simulink model "JIC"  (R2021b)
settings: Solver=ode3  StartTime=0.0  StopTime=10  FixedStep=.002  RelTol=1e-3  EnableMultiTasking=on
libraries: slpidlib x1
settings Model: ExtModeTrigDuration=10000  Creator=smascaro  LastModifiedBy=zorto
settings SolverCC: AlgebraicLoopSolver=TrustRegion  PositivePriorityOrder=on
settings DataIOCC: SaveFormat=Array  SignalLoggingSaveFormat=ModelDataLogs  SaveOutput=off  SaveTime=off  ReturnWorkspaceOutputs=off
settings OptimizationCC: ExpressionDepthLimit=2147483647  InitFltsAndDblsToZero=on  LifeSpan=inf
settings DebuggingCC: SaveWithParameterizedLinksMsg=none  UnderspecifiedInitializationDetection=Classic  MergeDetectMultiDrivingBlocksExec=none  SignalResolutionControl=TryResolveAllWithWarning  SolverPrmCheckMsg=warning  MultiTaskDSMMsg=warning  MultiTaskCondExecSysMsg=none  FcnCallInpInsideContextMsg=warning  AllowSymbolicDim=off  StateNameClashWarn=warning  SFUnexpectedBacktrackingDiag=warning  SFNoUnconditionalDefaultTransitionDiag=warning  SFExecutionAtInitializationDiag=none  SFMachineParentedDataDiag=warning  ArithmeticOperatorsInVariantConditions=warning
settings HardwareCC: ProdBitPerPointer=32  ProdBitPerSizeT=32  ProdBitPerPtrDiffT=32  ProdLargestAtomicFloat=None  ProdIntDivRoundTo=Undefined  ProdEndianess=Unspecified  ProdWordSize=32  ProdHWDeviceType=32-bit Generic  TargetBitPerPointer=64  TargetBitPerSizeT=64  TargetBitPerPtrDiffT=64  TargetLongLongMode=on  TargetIntDivRoundTo=Zero  TargetEndianess=LittleEndian  TargetWordSize=64  TargetHWDeviceType=MATLAB Host
settings ModelReferenceCC: PropagateSignalLabelsOutOfModel=off
settings SFSimCC: SimUseLocalCustomCode=off  SimParseCustomCode=off  CustomCodeUndefinedFunction=UseInterfaceOnly
settings RTWCC: Description=QUARC Win32 Target  SystemTargetFile=quarc_windows.tlc  TemplateMakefile=quarc_default_tmf  RTWUseLocalCustomCode=off
settings CodeAppCC: StateflowObjectComments=on
settings STFCustomTargetCC: TargetPreCompLibLocation=C:\PROGRA~3\QUARC\lib\2015b\windows\release  CPPClassGenCompliant=on  SystemTargetFile=quarc_windows.tlc
settings GRTTargetCC: TargetPreCompLibLocation=C:\PROGRA~3\QUARC\lib\2015b\windows\release  TargetLangStandard=C89/C90 (ANSI)  ParMdlRefBuildCompliant=off  CompOptLevelCompliant=off  ConcurrentExecutionCompliant=off  CombineOutputUpdateFcns=off  MatFileLogging=off  GRTInterface=on  UseToolchainInfoCompliant=off  ExtMode=on  ExtModeMexFile=quarc_comm
settings ConfigComp: CovMetricSettings=dw  CovSaveCumulativeToWorkspaceVar=on  CovSaveSingleToWorkspaceVar=on  CovExternalEMLEnable=off

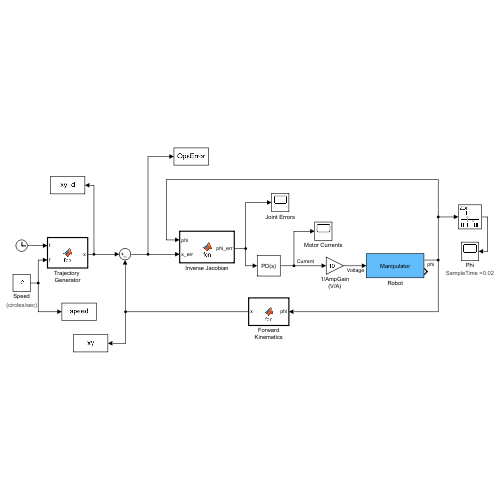
[thumbnail: Simulink's stored preview of the top-level diagram]
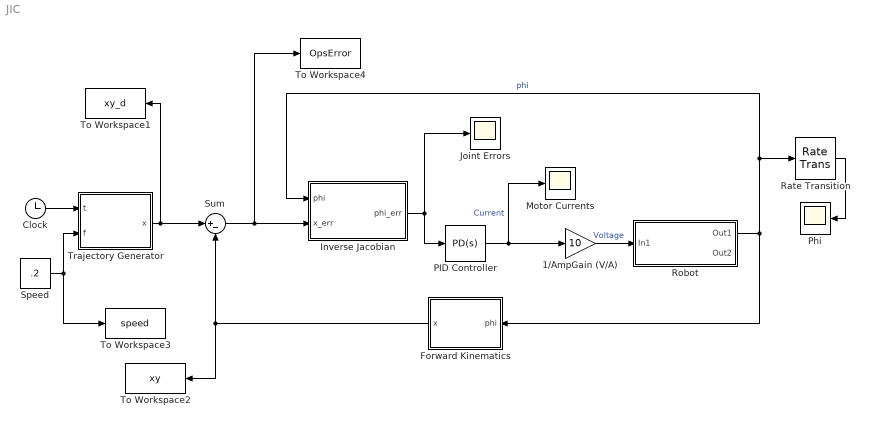
== system JIC ==
  1/AmpGain (V/A) : Gain  Gain=10
  Clock : Clock
  Forward Kinematics : MATLAB Function  TreatAsAtomicUnit=on
  Inverse Jacobian : MATLAB Function  TreatAsAtomicUnit=on
  Joint Errors : Scope
  Motor Currents : Scope
  PID Controller : slpidlib/PID Controller  Controller=PD  Form=Parallel  TimeDomain=Continuous-time  UseExternalTs=off  SampleTime=-1  IntegratorMethod=Forward Euler  FilterMethod=Forward Euler  ControllerParametersSource=internal  P=8  I=1  D=0.27  UseFilter=on  N=100  TunerSelectOption=Transfer Function Based (PID Tuner App)  InitialConditionSource=internal  InitialConditionForIntegrator=0  InitialConditionForFilter=0  DifferentiatorICPrevScaledInput=0  ExternalReset=none  TrackingMode=off  Kt=1  LimitOutput=off  SatLimitsSource=internal  UpperSaturationLimit=inf  LowerSaturationLimit=-inf  LinearizeAsGain=on  AntiWindupMode=none  Kb=1  POutMin=[]  POutMax=[]  IOutMin=[]  IOutMax=[]  DOutMin=[]  DOutMax=[]  NOutMin=[]  NOutMax=[]  SumOutMin=[]  SumOutMax=[]  SaturationOutMin=[]  SaturationOutMax=[]  PParamMin=[]  PParamMax=[]  IParamMin=[]  IParamMax=[]  DParamMin=[]  DParamMax=[]  NParamMin=[]  NParamMax=[]  KbParamMin=[]  KbParamMax=[]  KtParamMin=[]  KtParamMax=[]  KbOutMin=[]  KbOutMax=[]  KtOutMin=[]  KtOutMax=[]  IntegratorOutMin=[]  IntegratorOutMax=[]  FilterOutMin=[]  FilterOutMax=[]  SumI1OutMin=[]  SumI1OutMax=[]  SumI2OutMin=[]  SumI2OutMax=[]  SumI3OutMin=[]  SumI3OutMax=[]  SumI4OutMin=[]  SumI4OutMax=[]  SumDOutMin=[]  SumDOutMax=[]  DifferentiatorOutMin=[]  DifferentiatorOutMax=[]  FilterDiffOutCoefMin=[]  FilterDiffOutCoefMax=[]  ReciprocalOutMin=[]  ReciprocalOutMax=[]  SumDenOutMin=[]  SumDenOutMax=[]  SumNumOutMin=[]  SumNumOutMax=[]  DivideOutMin=[]  DivideOutMax=[]  UdiffTsProdOutMin=[]  UdiffTsProdOutMax=[]  NTsProdOutMin=[]  NTsProdOutMax=[]  UintegralTsProdOutMin=[]  UintegralTsProdOutMax=[]  UngainTsProdOutMin=[]  UngainTsProdOutMax=[]  IntegratorContinuousStateAttributes=''  IntegratorStateMustResolveToSignalObject=off  IntegratorRTWStateStorageClass=Auto  FilterContinuousStateAttributes=''  FilterStateMustResolveToSignalObject=off  FilterRTWStateStorageClass=Auto  ParallelPVariant=InternalParameters  IdealPVariant=Disabled  IVariant=Disabled  DVariant=InternalParameters  IntegratorVariant=Disabled  SatVariant=Disabled  AWVariant=Disabled  PCopyVariant=Disabled  TRVariant=Disabled  FdbkBlocksVariant=Forward  IdealPFdbkVariant=Disabled  SatFdbkVariant=Disabled  DerivativeFilterVariant=ContFilter  NVariant=InternalParameters  NCopyVariant=Disabled  FilterICVariant=InternalICsFilter  IntegratorICVariant=Disabled  ExternalResetVariant=Disabled  TRSumVariant=Passthrough  SumFdbkVariant=Disabled  SumVariant=Sum_PD  TsampFilterVariant=InternalTs  TsampNgainVariant=Passthrough  TsampIntegralVariant=Disabled_SignalSpec  ExternalSaturationOutDataTypeStr=Inherit: Same as second input
  Phi : Scope
      settings: AttributesFormatString=SampleTime =%<SampleTime>
  Rate Transition : RateTransition  OutPortSampleTimeOpt=Inherit  OutPortSampleTimeMultiple=10  OutPortSampleTime=0.05
  Robot : Subsystem
      mask Display: disp('Manipulator')
  Speed : Constant  Value=.2
      settings: AttributesFormatString=(circles/sec)
  Sum : Sum  Inputs=|+-
  To Workspace1 : ToWorkspace  VariableName=xy_d  SampleTime=-1
  To Workspace2 : ToWorkspace  VariableName=xy  SampleTime=-1
  To Workspace3 : ToWorkspace  VariableName=speed  SampleTime=-1
  To Workspace4 : ToWorkspace  VariableName=OpsError  SaveFormat=Structure With Time  SampleTime=-1
  Trajectory Generator : MATLAB Function  TreatAsAtomicUnit=on
  wires:
  Robot/1(Out1) -> Inverse Jacobian/1(phi), Rate Transition/1, Forward Kinematics/1(phi)  "phi"
  Trajectory Generator/1(x) -> Sum/1, To Workspace1/1
  Forward Kinematics/1(x) -> To Workspace2/1, Sum/2
  Clock/1 -> Trajectory Generator/1(t)
  Speed/1 -> Trajectory Generator/2(f), To Workspace3/1
  1/AmpGain (V/A)/1 -> Robot/1(In1)  "Voltage"
  PID Controller/1 -> Motor Currents/1, 1/AmpGain (V/A)/1  "Current"
  Rate Transition/1 -> Phi/1
  Sum/1 -> To Workspace4/1, Inverse Jacobian/2(x_err)
  Inverse Jacobian/1(phi_err) -> PID Controller/1, Joint Errors/1

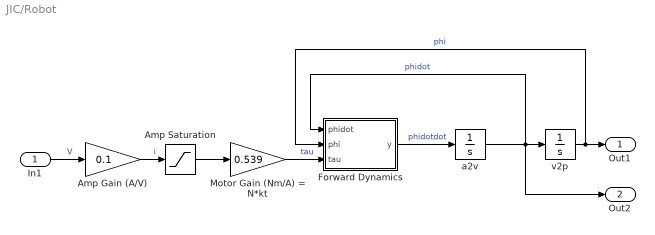
== system JIC/Robot ==
  In1 : Inport
  Amp Saturation : Saturate  UpperLimit=1  LowerLimit=-1  ZeroCross=off
  Amp Gain (A/V) : Gain  Gain=0.1
  Forward Dynamics : MATLAB Function  TreatAsAtomicUnit=on
  Motor Gain (Nm/A) = N*kt : Gain  Gain=0.539
  a2v : Integrator
  v2p : Integrator  InitialCondition=[1.1934;-0.2661]
  Out1 : Outport
  Out2 : Outport  Port=2
  wires:
  Forward Dynamics/1(y) -> a2v/1  "phidotdot"
  a2v/1 -> v2p/1, Out2/1, Forward Dynamics/1(phidot)  "phidot"
  v2p/1 -> Out1/1, Forward Dynamics/2(phi)  "phi"
  In1/1 -> Amp Gain (A/V)/1  "V"
  Motor Gain (Nm/A) = N*kt/1 -> Forward Dynamics/3(tau)  "tau"
  Amp Saturation/1 -> Motor Gain (Nm/A) = N*kt/1
  Amp Gain (A/V)/1 -> Amp Saturation/1  "i"

== matlab function JIC/Robot/Forward Dynamics ==
  settings: fimath=|
      | fimath(...
      | 'RoundMode', 'floor',...
      | 'OverflowMode', 'wrap',...
      | 'ProductMode', 'KeepLSB', 'ProductWordLength', 32,...
      | 'SumMode', 'KeepLSB', 'SumWordLength', 32,...
      | 'CastBeforeSum', false)
  data: phidot input double size=2; phi input double size=2; y output double size=2; tau input size=2
function y = fcn(phidot,phi,tau)
% This block supports an embeddable subset of the MATLAB language.
% See the help menu for details. 

a1 = 0.15;  % link 1 length
a2 = 0.15;  % link 2 length
m1 = 0.092;  % link 1 mass  
m2 = 0.077; % link 2 mas
r01 = 0.062; % link 1 center of mass
r12 = 0.036; % link 2 COM
I1 = 0.64e-3;  % link 1 inertia
I2 = 0.30e-3;  % link 2 inertia
Jm1 = 0.65e-6; % motor inertias
Jm2 = 0.65e-6;
b1 = 3.1e-6; % viscous damping constants
b2 = 3.1e-6;
c1 = 0.0001; % coulomb friction constants
c2 = 0.0001;
g = 9.8; % gravitational constant
N1 = 70; % gear ratios
N2 = 70;

H11 = N1^2*Jm1 + I1 + m2*a1^2;
H12 = a1*r12*m2*cos(phi(2)-phi(1));
H21 = H12;
H22 = N2^2*Jm2 + I2;
h = a1*r12*m2*sin(phi(2)-phi(1));
G1 = (r01*m1+a1*m2)*g*cos(phi(1));
G2 = r12*m2*g*cos(phi(2));
F1 = N1^2*b1*phidot(1) + N1*c1*sign(phidot(1));
F2 = N2^2*b2*phidot(2) + N2*c2*sign(phidot(2));

H = [H11 H12; H21 H22]; % inertia matrix
V = [0 -h ;h 0]*[phidot(1)^2;phidot(2)^2]; % centripetal torques
G = [G1;G2]; % gravity torques
F = [F1;F2]; % frictional torques

y = inv(H)*(tau - V - G - F); % y=phidotdot

== matlab function JIC/Forward Kinematics ==
  settings: fimath=|
      | fimath(...
      | 'RoundMode', 'floor',...
      | 'OverflowMode', 'wrap',...
      | 'ProductMode', 'KeepLSB', 'ProductWordLength', 32,...
      | 'SumMode', 'KeepLSB', 'SumWordLength', 32,...
      | 'CastBeforeSum', false)
  data: x output; phi input
function x = fcn(phi)
% This block supports an embeddable subset of the MATLAB language.
% See the help menu for details. 

a1=0.15;
a2=0.15;
x = [0;0];
x(1) = a1*cos(phi(1))+a2*cos(phi(2));
x(2) = a1*sin(phi(1))+a2*sin(phi(2));

== matlab function JIC/Trajectory Generator ==
  settings: fimath=|
      | fimath(...
      | 'RoundMode', 'floor',...
      | 'OverflowMode', 'wrap',...
      | 'ProductMode', 'KeepLSB', 'ProductWordLength', 32,...
      | 'SumMode', 'KeepLSB', 'SumWordLength', 32,...
      | 'CastBeforeSum', false)
  data: x output; t input; f input
function x = fcn(t,f)
% This block supports an embeddable subset of the MATLAB language.
% See the help menu for details. 
x = [0;0];

if t<0.5  % accelerate into circling trajectory
    x(1) = 0.075*cos(2*pi*f*t^2) + 0.125;
    x(2) = 0.075*sin(2*pi*f*t^2) + 0.1;
else  % constant speed circling of radius 0.075 about x=[0.125,0.1]
    x(1) = 0.075*cos(2*pi*f*(t-0.25)) + 0.125;
    x(2) = 0.075*sin(2*pi*f*(t-0.25)) + 0.1;
end

== matlab function JIC/Inverse Jacobian ==
  settings: fimath=|
      | fimath(...
      | 'RoundMode', 'floor',...
      | 'OverflowMode', 'wrap',...
      | 'ProductMode', 'KeepLSB', 'ProductWordLength', 32,...
      | 'SumMode', 'KeepLSB', 'SumWordLength', 32,...
      | 'CastBeforeSum', false)
  data: phi input; phi_err output; x_err input
function phi_err = fcn(phi, x_err)
%Inverse jacobian 
a1=0.15;
a2=0.15;

J =[-a1*sin(phi(1)) - a2*sin(phi(2)), -a2*sin(phi(2)) ; a1*cos(phi(1)) + a2*cos(phi(2)), a2*cos(phi(2))] *[1, 0 ; -1, 1];

Jinv = inv(J);

phi_err = Jinv * x_err;
